simulink library "robotlib"  (R2025a)
settings: Solver=ode45  StartTime=0.0  StopTime=10.0  RelTol=1e-3  EnableMultiTasking=on
undefined symbols (not defined in the file): coder, Count, Data, Data_SL_Info, Datatype, Encoding, Encoding_SL_Info, Fields, Fields_SL_Info, Header, Height, Name, Name_SL_Info, Offset, PointStep, ros, RowStep, Step, Width
libraries: $bdroot x1
(part 2 of 2)

== matlab function robotlib/Write Image/MATLAB Function ==
  data: Data input; Image input; Alpha input; unused input; Data output; Height output; Width output; DataLength output; Encoding output; EncodingLength output; Step output; EncodingStruct parameter; ImageEncoding parameter; HasAlpha parameter
function [Data, Height, Width, DataLength, Encoding, EncodingLength, Step]...
    = WriteImageFcnBlock(Data, Image, Alpha, ~, EncodingStruct, ImageEncoding, HasAlpha)
SelectedEncodingInd = ImageEncoding;
% Image encoding is set to evaluate in the mask,
% so the value is an index.
SelectedEncoding = ros.msg.sensor_msgs.internal.ImageEncoding.AllEncodings{SelectedEncodingInd};
type = EncodingStruct.DataType;
alphaSize = int32(size(Alpha));
imageSize = int32(size(Image));
% check types
if HasAlpha && ~isa(Alpha, type)
coder.internal.error('ros:slros:image:InvalidAlphaType', SelectedEncoding, type)
elseif HasAlpha && ~ismatrix(Alpha)
coder.internal.error('ros:slros:image:InvalidAlphaSize')
elseif ~isa(Image, type)
coder.internal.error('ros:slros:image:InvalidImageType', SelectedEncoding, type)
end
if HasAlpha
    % check sizes
    if ~(imageSize(1) == alphaSize(1) && imageSize(2) == alphaSize(2))
        coder.internal.error('ros:slros:image:IncompatibleImageAlphaSizes', ...
        fprintf("[%i, %i, %i]", imageSize(1), imageSize(2), imageSize(3)), ...
        fprintf("[%i, %i]", alphaSize(1), alphaSize(2)) )
    end

    ImageInput = cat(3, Image, Alpha);
else
    ImageInput = Image;
end
[Data, Height, Width, DataLength, Encoding, EncodingLength, Step]...
    = ros.internal.block.WriteImageFcnBlock(ImageInput, Data, EncodingStruct, SelectedEncodingInd);
